simulink model "wrm_r1"  (R2015a)
settings: Solver=ode45  StartTime=0.0  StopTime=10.0  RelTol=1e-3
settings Model: Creator=rojas-j  LastModifiedBy=rojas-j

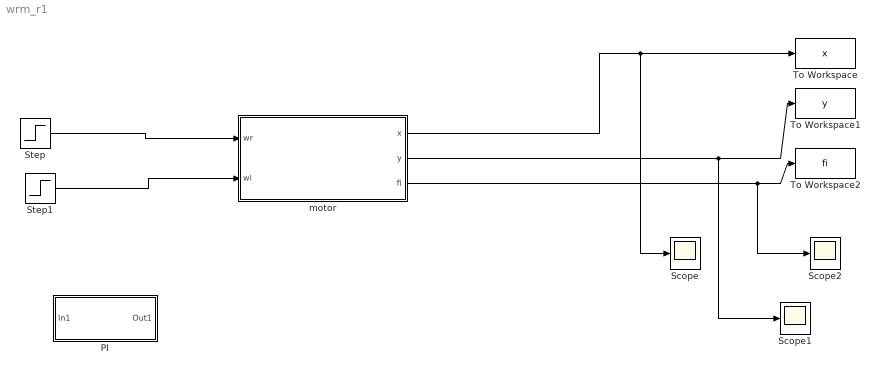
== system wrm_r1 ==
  PI : Subsystem
  Scope : Scope
  Scope1 : Scope
  Scope2 : Scope
      settings: SaveName=ScopeData2
  Step : Step  SampleTime=0
  Step1 : Step  After=-1  SampleTime=0
  To Workspace : ToWorkspace  VariableName=x  SaveFormat=Timeseries  SampleTime=-1
  To Workspace1 : ToWorkspace  VariableName=y  SaveFormat=Timeseries  SampleTime=-1
  To Workspace2 : ToWorkspace  VariableName=fi  SaveFormat=Timeseries  SampleTime=-1
  motor : Subsystem
  wires:
  motor/1(x) -> Scope/1, To Workspace/1
  motor/2(y) -> Scope1/1, To Workspace1/1
  motor/3(fi) -> Scope2/1, To Workspace2/1
  Step/1 -> motor/1(wr)
  Step1/1 -> motor/2(wl)

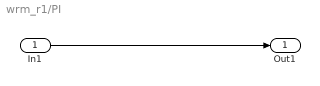
== system wrm_r1/PI ==
  In1 : Inport
  Out1 : Outport
  wires:
  In1/1 -> Out1/1

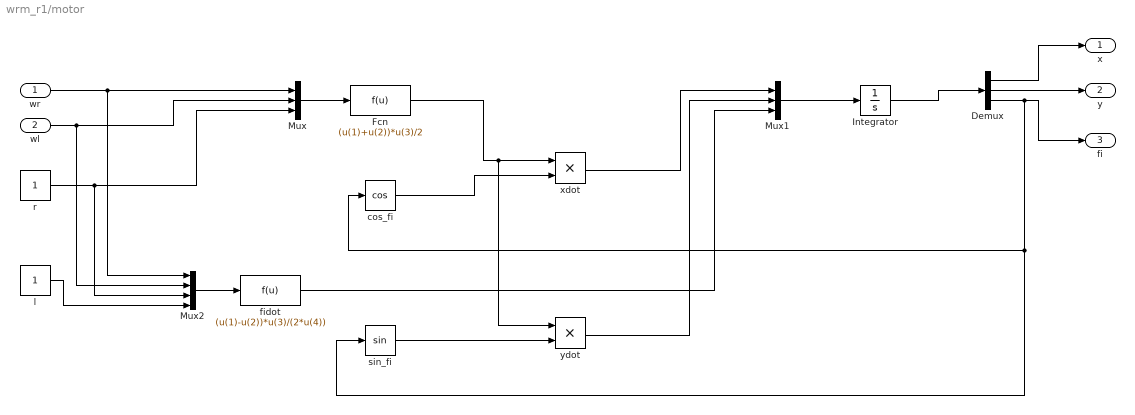
== system wrm_r1/motor ==
  wr : Inport
  wl : Inport  Port=2
  Demux : Demux  Outputs=3
  Fcn : Fcn  Expr=(u(1)+u(2))*u(3)/2
  Integrator : Integrator
  Mux : Mux  Inputs=3
  Mux1 : Mux  Inputs=3
  Mux2 : Mux
  "cos_fi " : Trigonometry  Operator=cos
  fidot : Fcn  Expr=(u(1)-u(2))*u(3)/(2*u(4))
  l : Constant
  r : Constant
  "sin_fi " : Trigonometry
  xdot : Product
  ydot : Product
  x : Outport
  y : Outport  Port=2
  fi : Outport  Port=3
  wires:
  wr/1 -> Mux2/1, Mux/1
  wl/1 -> Mux2/2, Mux/2
  Mux/1 -> Fcn/1
  Mux1/1 -> Integrator/1
  Integrator/1 -> Demux/1
  Demux/1 -> x/1
  Demux/2 -> y/1
  Demux/3 -> "sin_fi "/1, "cos_fi "/1, fi/1
  Fcn/1 -> ydot/1, xdot/1
  "cos_fi "/1 -> xdot/2
  xdot/1 -> Mux1/1
  "sin_fi "/1 -> ydot/2
  r/1 -> Mux2/3, Mux/3
  ydot/1 -> Mux1/2
  Mux2/1 -> fidot/1
  l/1 -> Mux2/4
  fidot/1 -> Mux1/3
